simulink model "IEEE123bus_v2019b_Discrete"  (R2019b)
(part 2 of 7)

  97/RConn3 -- 97-1/LConn3 -- 97-98 3/LConn3
  97-98 3/LConn2 -- 97-1/LConn2 -- 97/RConn2
  197/RConn1 -- 197-101 3/LConn1
  99/RConn3 -- 99-100 3/LConn3
  86/LConn3 -- 76-86 3/RConn3
  79 Y Z/LConn1 -- Load Flow Bus117/LConn1 -- 79/RConn1
  78-80 6/LConn2 -- 78/RConn2 -- 78-79 6/LConn2
  80/LConn1 -- 78-80 6/RConn1
